simulink model "Model_1_PI_Gain_TestBench"  (R2021a)
settings: Solver=VariableStepAuto  StartTime=0.0  StopTime=5  MaxStep=1e-4  RelTol=1e-3  EnableMultiTasking=on
values from neighbouring files (symbols this model uses):
  Gain_I = 26    [Model_1_Initialization.m]
  Gain_P = 7    [Model_1_Initialization.m]
  Id_reference = 0    [Model_1_Initialization.m]
  Iq_reference = 100    [Model_1_Initialization.m]
  Lambda_m = 0.2205    [Model_1_Initialization.m]
  Ld = 1.7e-3    (= 0.0017)    [Model_1_Initialization.m]
  Lq = 3.2e-3    (= 0.0032)    [Model_1_Initialization.m]
  Polepairs = 4    [Model_1_Initialization.m]
  Rs = 0.02    [Model_1_Initialization.m]
libraries: spsSVPWMGenerator2LevelLib x6, spsControlledVoltageSourceLib x3, spsVoltageMeasurementLib x3, pid_lib x2, spsPermanentMagnetSynchronousMachineLib x1, spsGroundLib x1, spspowerguiLib x1
settings Model: Creator=dakaihu  LastModifiedBy=Hidayet
settings SolverCC: AlgebraicLoopSolver=TrustRegion
settings DataIOCC: LimitDataPoints=on  ReturnWorkspaceOutputs=off
settings OptimizationCC: LifeSpan=inf
settings DebuggingCC: AllowSymbolicDim=off  SFUnexpectedBacktrackingDiag=warning  SFNoUnconditionalDefaultTransitionDiag=warning  SFExecutionAtInitializationDiag=none  SFMachineParentedDataDiag=warning  ArithmeticOperatorsInVariantConditions=warning
settings ModelReferenceCC: PropagateSignalLabelsOutOfModel=off
settings SFSimCC: SimUseLocalCustomCode=off  CustomCodeUndefinedFunction=UseInterfaceOnly
settings RTWCC: RTWUseLocalCustomCode=off
settings CodeAppCC: StateflowObjectComments=on
settings GRTTargetCC: TargetLangStandard=C89/C90 (ANSI)
settings ConfigComp: CovMetricSettings=dw  CovSaveCumulativeToWorkspaceVar=on  CovSaveSingleToWorkspaceVar=on  CovExternalEMLEnable=off
settings SimscapeCC: SimscapeNormalizeSystem=off

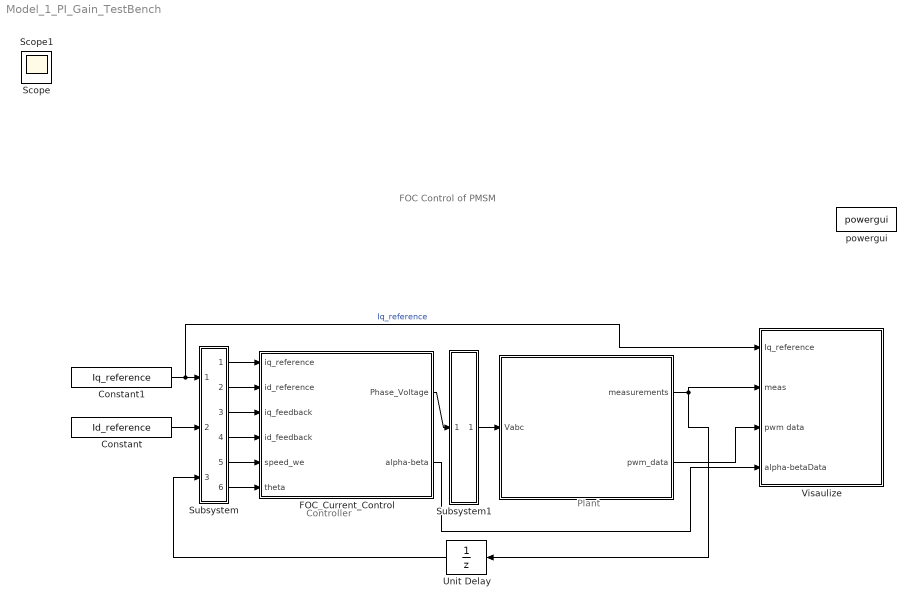
== system Model_1_PI_Gain_TestBench ==
  note: Controller
  note: Plant
  note: FOC Control of PMSM
  " " : Subsystem
  Constant : Constant  Value=Id_reference
  Constant1 : Constant  Value=Iq_reference  VectorParams1D=off
  FOC_Current_Control : Subsystem
  Subsystem : Subsystem
      mask Display: fprintf('C/D')
  Subsystem1 : Subsystem
      mask Display: fprintf('D/C')
  Unit Delay : UnitDelay  SampleTime=1e-4  HasFrameUpgradeWarning=on
  Visaulize : Subsystem
  powergui : spspowerguiLib/powergui  SimulationMode=Continuous  SampleTime=1e-5  frequency=60  Iterations=50  frequencyindice=0  Pbase=100e6  ErrMax=1e-4  UnitsV=kV  UnitsW=MW  buscounter=0  FunctionMessages=off  echomessages=off  EnableUseOfTLC=off  CurrentSourceSwitches=off  DisableSnubberDevices=off  DisableRonSwitches=off  DisableVfSwitches=off  DisplayEquations=off  AutomaticDiscreteSolvers=off  SolverType=Tustin/Backward Euler (TBE)  Interpol=off  ExternalGateDelay=off  methode=off  Ts=100  x0status=blocks  SPID=on  SwTol=0  HookPort=off  NonlinearTolerance=1e-4  nMaxIteration=100  ContinueOnMaxIteration=off  RestoreLinks=warning  ResistiveCurrentMeasurement=off  Frange=[0:2:500]  Ylog=off  Xlog=on  ShowGrid=off  save=off  variable=ZData  structure=0  ZoomFFT=on  StartTime=0.0  cycles=1  DisplayStyle=1  fundamental=60  FreqAxis=off  MaxFrequency=1000  frequencyindicesteady=1  RmsSteady=1  display=off
  Scope : Scope
  Scope1 : Scope
  wires:
  FOC_Current_Control/1(Phase_Voltage) -> Subsystem1/1(In1)
  " "/1(measurements) -> Unit Delay/1, Visaulize/2(meas)
  Subsystem/3(Out2) -> FOC_Current_Control/3(iq_feedback)
  Subsystem/4(Out3) -> FOC_Current_Control/4(id_feedback)
  Subsystem1/1(Out1) -> " "/1(Vabc)
  Unit Delay/1 -> Subsystem/3(PMSM_Measurements)
  Subsystem/5(Out1) -> FOC_Current_Control/5(speed_we)
  Subsystem/6(Out4) -> FOC_Current_Control/6(theta)
  Constant/1 -> Subsystem/2(id_ref)
  Constant1/1 -> Visaulize/1(Iq_reference), Subsystem/1(iq_ref)  "Iq_reference"
  Subsystem/1(Out6) -> FOC_Current_Control/1(iq_reference)
  Subsystem/2(Out5) -> FOC_Current_Control/2(id_reference)
  FOC_Current_Control/2(alpha-beta) -> Visaulize/4(alpha-betaData)
  " "/2(pwm_data) -> Visaulize/3(pwm data)

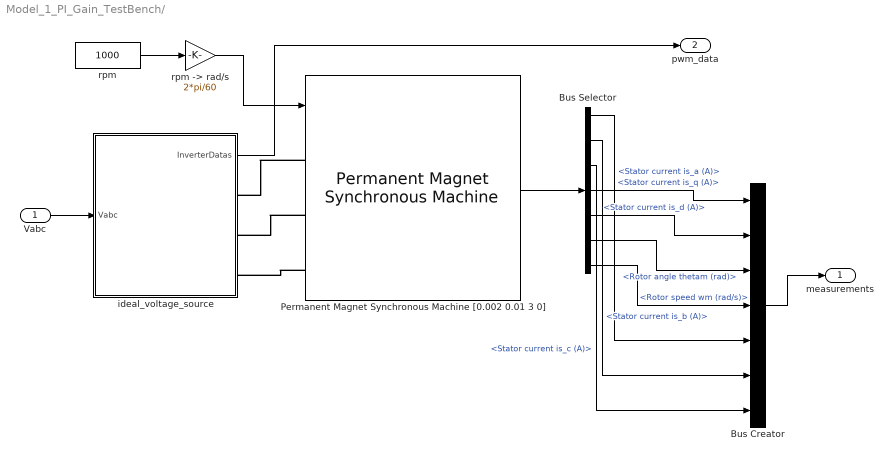
== system Model_1_PI_Gain_TestBench/  ==
  Vabc : Inport
  Bus Creator : BusCreator  Inputs=7
  Bus Selector : BusSelector  OutputSignals=Stator current is_a (A),Stator current is_b (A),Stator current is_c (A),Stator current is_q (A),Stator current is_d (A),Rotor angle thetam (rad),Rotor speed wm (rad/s)
  Permanent Magnet Synchronous Machine [0.002 0.01 3 0] : spsPermanentMagnetSynchronousMachineLib/Permanent Magnet Synchronous Machine  NbPhases=3  FluxDistribution=Sinusoidal  RotorType=Salient-pole  MechanicalLoad=Speed w  PresetModel=No  ShowDetailedParameters=on  MeasurementBus=off  Resistance=Rs  Inductance=8.5e-3  dqInductances=[Ld,Lq]  La=0.000395  MachineConstant=Flux linkage established by magnets (V.s)  Flux=Lambda_m  VoltageCst=159.9771  TorqueCst=1.323  Flat=120  Mechanical=[0.0027 0.001 4 0]  PolePairs=Polepairs  InitialConditions=[0,0, 0,0]  InitialConditions5ph=[0 0 0 0 0 0]  RefAngle=Aligned with phase A axis (original Park)  IterativeDiscreteModel=Trapezoidal non iterative  TsBlock=-1  TsPowergui=0
  ideal_voltage_source : Subsystem  VariantControl=variantPwm == enumPwm.behavior
  rpm : Constant  Value=1000
  "rpm -> rad/s" : Gain  Gain=2*pi/60
  measurements : Outport  VectorParamsAs1DForOutWhenUnconnected=off
  pwm_data : Outport  Port=2
  wires:
  Vabc/1 -> ideal_voltage_source/1(Vabc)
  rpm/1 -> "rpm -> rad/s"/1
  Bus Selector/4 -> Bus Creator/1  "<Stator current is_q (A)>"
  Bus Selector/5 -> Bus Creator/2  "<Stator current is_d (A)>"
  Bus Selector/6 -> Bus Creator/3  "<Rotor angle thetam (rad)>"
  Bus Creator/1 -> measurements/1
  Bus Selector/1 -> Bus Creator/5  "<Stator current is_a (A)>"
  Bus Selector/2 -> Bus Creator/6  "<Stator current is_b (A)>"
  Bus Selector/3 -> Bus Creator/7  "<Stator current is_c (A)>"
  Permanent Magnet Synchronous Machine [0.002 0.01 3 0]/1 -> Bus Selector/1
  Bus Selector/7 -> Bus Creator/4  "<Rotor speed wm (rad/s)>"
  "rpm -> rad/s"/1 -> Permanent Magnet Synchronous Machine [0.002 0.01 3 0]/1
  ideal_voltage_source/1(InverterDatas) -> pwm_data/1
  connections:
  Permanent Magnet Synchronous Machine [0.002 0.01 3 0]/LConn1 -- ideal_voltage_source/RConn1
  Permanent Magnet Synchronous Machine [0.002 0.01 3 0]/LConn2 -- ideal_voltage_source/RConn2
  Permanent Magnet Synchronous Machine [0.002 0.01 3 0]/LConn3 -- ideal_voltage_source/RConn3

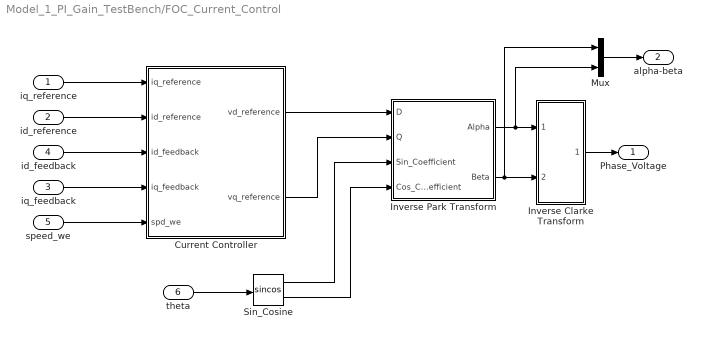
== system Model_1_PI_Gain_TestBench/FOC_Current_Control ==
  iq_reference : Inport  SampleTime=1e-4
  id_reference : Inport  Port=2  SampleTime=1e-4
  iq_feedback : Inport  Port=3  SampleTime=1e-4
  id_feedback : Inport  Port=4  SampleTime=1e-4
  speed_we : Inport  Port=5  SampleTime=1e-4
  theta : Inport  Port=6  SampleTime=1e-4
  Current Controller : Subsystem
  Inverse Clarke Transform : Subsystem
  Inverse Park Transform : Subsystem
  Mux : Mux  Inputs=2
  Sin_Cosine : Trigonometry  Operator=sincos
  Phase_Voltage : Outport  SampleTime=1e-4  VectorParamsAs1DForOutWhenUnconnected=off
  alpha-beta : Outport  Port=2
  wires:
  Inverse Clarke Transform/1(ABC) -> Phase_Voltage/1
  Sin_Cosine/2 -> Inverse Park Transform/4(Cos_Coefficient)
  Sin_Cosine/1 -> Inverse Park Transform/3(Sin_Coefficient)
  theta/1 -> Sin_Cosine/1
  Current Controller/2(vq_reference) -> Inverse Park Transform/2(Q)
  Current Controller/1(vd_reference) -> Inverse Park Transform/1(D)
  id_feedback/1 -> Current Controller/3(id_feedback)
  iq_feedback/1 -> Current Controller/4(iq_feedback)
  speed_we/1 -> Current Controller/5(spd_we)
  iq_reference/1 -> Current Controller/1(iq_reference)
  id_reference/1 -> Current Controller/2(id_reference)
  Mux/1 -> alpha-beta/1
  Inverse Park Transform/1(Alpha) -> Mux/2, Inverse Clarke Transform/1(Alpha)
  Inverse Park Transform/2(Beta) -> Mux/1, Inverse Clarke Transform/2(Beta)

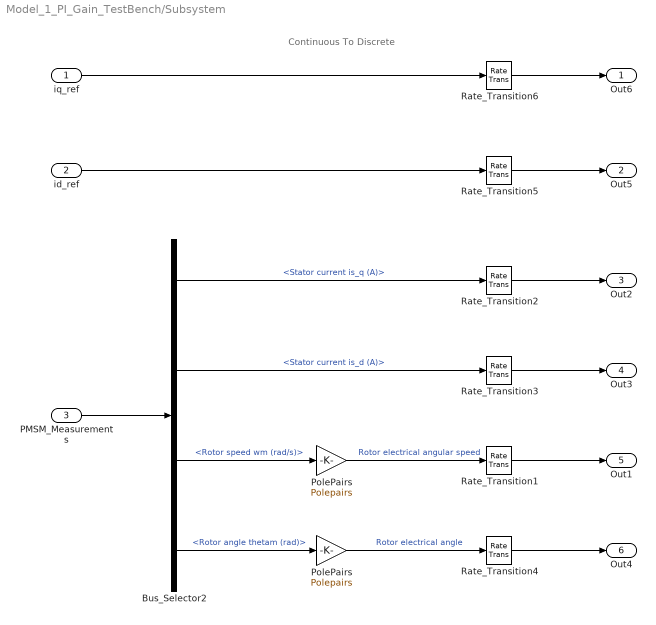
== system Model_1_PI_Gain_TestBench/Subsystem ==
  note: Continuous To Discrete
  iq_ref : Inport
  id_ref : Inport  Port=2
  PMSM_Measurements : Inport  Port=3
  Bus_Selector2 : BusSelector  OutputSignals=Stator current is_q (A),Stator current is_d (A),Rotor speed wm (rad/s),Rotor angle thetam (rad)
  PolePairs : Gain  Gain=Polepairs
  "PolePairs " : Gain  Gain=Polepairs
  Rate_Transition{1..6} (6 alike) : RateTransition  Integrity=off  Deterministic=off
  Out6 : Outport  VectorParamsAs1DForOutWhenUnconnected=off
  Out5 : Outport  Port=2  VectorParamsAs1DForOutWhenUnconnected=off
  Out2 : Outport  Port=3  VectorParamsAs1DForOutWhenUnconnected=off
  Out3 : Outport  Port=4  VectorParamsAs1DForOutWhenUnconnected=off
  Out1 : Outport  Port=5  VectorParamsAs1DForOutWhenUnconnected=off
  Out4 : Outport  Port=6  VectorParamsAs1DForOutWhenUnconnected=off
  wires:
  Rate_Transition4/1 -> Out4/1
  Bus_Selector2/2 -> Rate_Transition3/1  "<Stator current is_d (A)>"
  id_ref/1 -> Rate_Transition5/1
  iq_ref/1 -> Rate_Transition6/1
  Bus_Selector2/1 -> Rate_Transition2/1  "<Stator current is_q (A)>"
  Bus_Selector2/4 -> PolePairs/1  "<Rotor angle thetam (rad)>"
  PMSM_Measurements/1 -> Bus_Selector2/1
  PolePairs/1 -> Rate_Transition4/1  "Rotor electrical angle"
  Rate_Transition5/1 -> Out5/1
  Rate_Transition6/1 -> Out6/1
  Rate_Transition2/1 -> Out2/1
  Rate_Transition3/1 -> Out3/1
  Rate_Transition1/1 -> Out1/1
  Bus_Selector2/3 -> "PolePairs "/1  "<Rotor speed wm (rad/s)>"
  "PolePairs "/1 -> Rate_Transition1/1  "Rotor electrical angular speed"

== system Model_1_PI_Gain_TestBench/Subsystem1 ==
  In1 : Inport
  Rate_Transition1 : RateTransition  Integrity=off
  Out1 : Outport  VectorParamsAs1DForOutWhenUnconnected=off
  wires:
  In1/1 -> Rate_Transition1/1
  Rate_Transition1/1 -> Out1/1

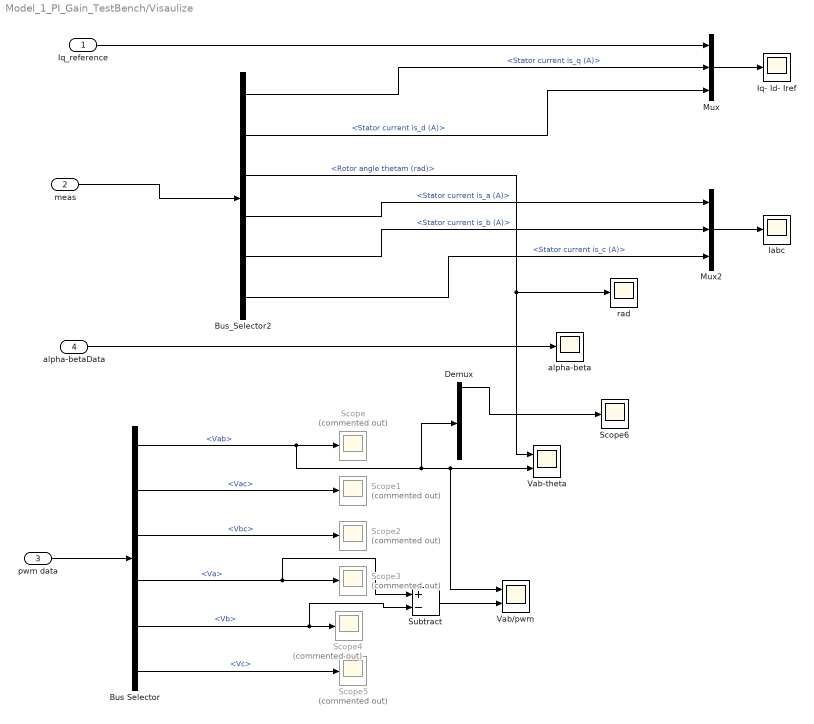
== system Model_1_PI_Gain_TestBench/Visaulize ==
  Iq_reference : Inport
  meas : Inport  Port=2
  pwm data : Inport  Port=3
  alpha-betaData : Inport  Port=4
  Bus Selector : BusSelector  OutputSignals=Vab,Vac,Vbc,Va,Vb,Vc
  Bus_Selector2 : BusSelector  OutputSignals=Stator current is_q (A),Stator current is_d (A),Rotor angle thetam (rad),Stator current is_a (A),Stator current is_b (A),Stator current is_c (A)
  Demux : Demux  Outputs=6
  Iabc : Scope
  Iq- Id- Iref : Scope
  Mux : Mux  Inputs=3
  Mux2 : Mux  Inputs=3
  Scope{,1..5} (6 alike) : Scope  Commented=on
  Scope6 : Scope
  Subtract : Sum  Inputs=+-
  Vab-theta : Scope  NumInputPorts=2
  Vab/pwm : Scope  NumInputPorts=2
  alpha-beta : Scope
  rad : Scope
  wires:
  meas/1 -> Bus_Selector2/1
  Mux/1 -> Iq- Id- Iref/1
  Bus_Selector2/2 -> Mux/3  "<Stator current is_d (A)>"
  Iq_reference/1 -> Mux/1
  Bus_Selector2/1 -> Mux/2  "<Stator current is_q (A)>"
  Mux2/1 -> Iabc/1
  alpha-betaData/1 -> alpha-beta/1
  Bus_Selector2/3 -> Vab-theta/1, rad/1  "<Rotor angle thetam (rad)>"
  pwm data/1 -> Bus Selector/1
  Bus Selector/1 -> Demux/1, Vab/pwm/1, Vab-theta/2, Scope/1  "<Vab>"
  Bus Selector/2 -> Scope1/1  "<Vac>"
  Bus Selector/3 -> Scope2/1  "<Vbc>"
  Bus Selector/4 -> Subtract/1, Scope3/1  "<Va>"
  Bus Selector/5 -> Subtract/2, Scope4/1  "<Vb>"
  Subtract/1 -> Vab/pwm/2
  Bus Selector/6 -> Scope5/1  "<Vc>"
  Bus_Selector2/4 -> Mux2/1  "<Stator current is_a (A)>"
  Bus_Selector2/5 -> Mux2/2  "<Stator current is_b (A)>"
  Bus_Selector2/6 -> Mux2/3  "<Stator current is_c (A)>"
  Demux/1 -> Scope6/1

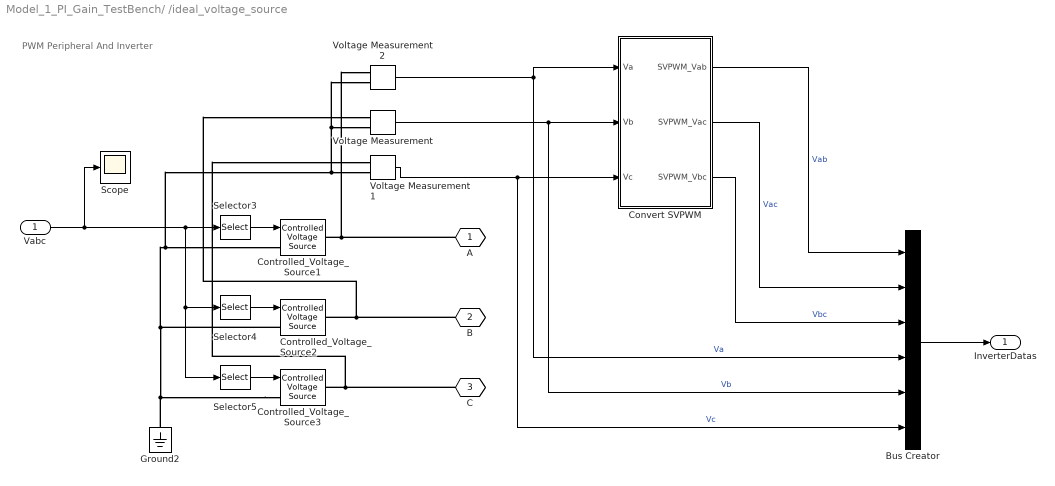
== system Model_1_PI_Gain_TestBench/ /ideal_voltage_source ==
  note: PWM Peripheral And Inverter
  Vabc : Inport
  Bus Creator : BusCreator  Inputs=6
  Controlled_Voltage_Source1 : spsControlledVoltageSourceLib/Controlled Voltage Source  Initialize=off  Source_Type=DC  Amplitude=12  Phase=0  Frequency=0  Measurements=None
  Controlled_Voltage_Source2 : spsControlledVoltageSourceLib/Controlled Voltage Source  Initialize=off  Source_Type=DC  Amplitude=12  Phase=0  Frequency=0  Measurements=None
  Controlled_Voltage_Source3 : spsControlledVoltageSourceLib/Controlled Voltage Source  Initialize=off  Source_Type=DC  Amplitude=12  Phase=0  Frequency=0  Measurements=None
  Convert SVPWM : Subsystem
  Ground2 : spsGroundLib/Ground  LConnTagsString=a
  Scope : Scope
  Selector3 : Selector  InputPortWidth=3  IndexOptions=Index vector (dialog)  Indices=[1]  OutputSizes=1
  Selector4 : Selector  InputPortWidth=3  IndexOptions=Index vector (dialog)  Indices=2  OutputSizes=1
  Selector5 : Selector  InputPortWidth=3  IndexOptions=Index vector (dialog)  Indices=3  OutputSizes=1
  Voltage Measurement : spsVoltageMeasurementLib/Voltage Measurement  PhasorSimulation=off  OutputType=Complex  PSBequivalent=0
  Voltage Measurement1 : spsVoltageMeasurementLib/Voltage Measurement  PhasorSimulation=off  OutputType=Complex  PSBequivalent=0
  Voltage Measurement2 : spsVoltageMeasurementLib/Voltage Measurement  PhasorSimulation=off  OutputType=Complex  PSBequivalent=0
  A : PMIOPort  Tag=PMCPort  Side=Right
  B : PMIOPort  Tag=PMCPort  Port=2  Side=Right
  C : PMIOPort  Tag=PMCPort  Port=3  Side=Right
  InverterDatas : Outport
  wires:
  Vabc/1 -> Scope/1, Selector4/1, Selector5/1, Selector3/1
  Selector5/1 -> Controlled_Voltage_Source3/1
  Selector4/1 -> Controlled_Voltage_Source2/1
  Selector3/1 -> Controlled_Voltage_Source1/1
  Voltage Measurement2/1 -> Bus Creator/4, Convert SVPWM/1(Va)  "Va"
  Voltage Measurement/1 -> Bus Creator/5, Convert SVPWM/2(Vb)  "Vb"
  Voltage Measurement1/1 -> Bus Creator/6, Convert SVPWM/3(Vc)  "Vc"
  Convert SVPWM/1(SVPWM_Vab) -> Bus Creator/1  "Vab"
  Convert SVPWM/2(SVPWM_Vac) -> Bus Creator/2  "Vac"
  Convert SVPWM/3(SVPWM_Vbc) -> Bus Creator/3  "Vbc"
  Bus Creator/1 -> InverterDatas/1
  connections:
  C/RConn1 -- Voltage Measurement1/LConn1 -- Controlled_Voltage_Source3/RConn1
  B/RConn1 -- Voltage Measurement/LConn1 -- Controlled_Voltage_Source2/RConn1
  A/RConn1 -- Voltage Measurement2/LConn1 -- Controlled_Voltage_Source1/RConn1
  Controlled_Voltage_Source3/LConn1 -- Voltage Measurement2/LConn2 -- Voltage Measurement/LConn2 -- Voltage Measurement1/LConn2 -- Controlled_Voltage_Source1/LConn1 -- Controlled_Voltage_Source2/LConn1 -- Ground2/LConn1

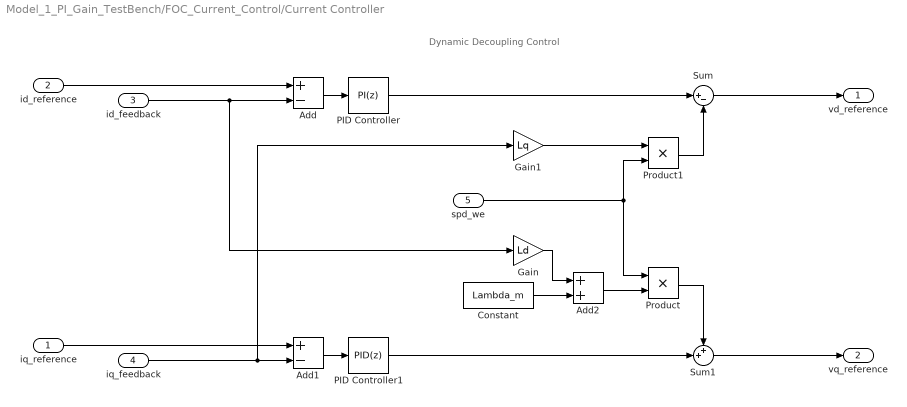
== system Model_1_PI_Gain_TestBench/FOC_Current_Control/Current Controller ==
  note: Dynamic Decoupling Control
  iq_reference : Inport  SampleTime=1e-4
  id_reference : Inport  Port=2  SampleTime=1e-4
  id_feedback : Inport  Port=3  SampleTime=1e-4
  iq_feedback : Inport  Port=4  SampleTime=1e-4
  spd_we : Inport  Port=5  SampleTime=1e-4
  Add : Sum  Inputs=+-
  Add1 : Sum  Inputs=+-
  Add2 : Sum
  Constant : Constant  Value=Lambda_m  SampleTime=1e-4
  Gain : Gain  Gain=Ld
  Gain1 : Gain  Gain=Lq
  PID Controller : pid_lib/PID Controller  Controller=PI  Form=Parallel  TimeDomain=Discrete-time  UseExternalTs=off  SampleTime=-1  IntegratorMethod=Forward Euler  FilterMethod=Forward Euler  ControllerParametersSource=internal  P=Gain_P  I=Gain_I  D=0  UseFilter=on  N=100  TunerSelectOption=Transfer Function Based (PID Tuner App)  InitialConditionSource=internal  InitialConditionForIntegrator=0  InitialConditionForFilter=0  DifferentiatorICPrevScaledInput=0  ExternalReset=none  TrackingMode=off  Kt=1  LimitOutput=off  SatLimitsSource=internal  UpperSaturationLimit=inf  LowerSaturationLimit=-inf  LinearizeAsGain=on  AntiWindupMode=none  Kb=1  POutMin=[]  POutMax=[]  IOutMin=[]  IOutMax=[]  DOutMin=[]  DOutMax=[]  NOutMin=[]  NOutMax=[]  SumOutMin=[]  SumOutMax=[]  SaturationOutMin=[]  SaturationOutMax=[]  PParamMin=[]  PParamMax=[]  IParamMin=[]  IParamMax=[]  DParamMin=[]  DParamMax=[]  NParamMin=[]  NParamMax=[]  KbParamMin=[]  KbParamMax=[]  KtParamMin=[]  KtParamMax=[]  KbOutMin=[]  KbOutMax=[]  KtOutMin=[]  KtOutMax=[]  IntegratorOutMin=[]  IntegratorOutMax=[]  FilterOutMin=[]  FilterOutMax=[]  SumI1OutMin=[]  SumI1OutMax=[]  SumI2OutMin=[]  SumI2OutMax=[]  SumI3OutMin=[]  SumI3OutMax=[]  SumI4OutMin=[]  SumI4OutMax=[]  SumDOutMin=[]  SumDOutMax=[]  DifferentiatorOutMin=[]  DifferentiatorOutMax=[]  FilterDiffOutCoefMin=[]  FilterDiffOutCoefMax=[]  ReciprocalOutMin=[]  ReciprocalOutMax=[]  SumDenOutMin=[]  SumDenOutMax=[]  SumNumOutMin=[]  SumNumOutMax=[]  DivideOutMin=[]  DivideOutMax=[]  UdiffTsProdOutMin=[]  UdiffTsProdOutMax=[]  NTsProdOutMin=[]  NTsProdOutMax=[]  UintegralTsProdOutMin=[]  UintegralTsProdOutMax=[]  UngainTsProdOutMin=[]  UngainTsProdOutMax=[]  IntegratorContinuousStateAttributes=''  IntegratorStateMustResolveToSignalObject=off  IntegratorRTWStateStorageClass=Auto  FilterContinuousStateAttributes=''  FilterStateMustResolveToSignalObject=off  FilterRTWStateStorageClass=Auto  ParallelPVariant=InternalParameters  IdealPVariant=Disabled  IVariant=InternalParameters  DVariant=Disabled  IntegratorVariant=Discrete  SatVariant=Disabled  AWVariant=Passthrough  PCopyVariant=Disabled  TRVariant=Disabled  FdbkBlocksVariant=Forward  IdealPFdbkVariant=Disabled  SatFdbkVariant=Disabled  DerivativeFilterVariant=Disabled  NVariant=Disabled  NCopyVariant=Disabled_SignalSpec  FilterICVariant=Disabled  IntegratorICVariant=InternalICs  ExternalResetVariant=Disabled  TRSumVariant=Passthrough  SumFdbkVariant=Disabled  SumVariant=Sum_PI  TsampFilterVariant=InternalTs  TsampNgainVariant=Passthrough  TsampIntegralVariant=Passthrough  ExternalSaturationOutDataTypeStr=Inherit: Same as second input
  PID Controller1 : pid_lib/PID Controller  Controller=PID  Form=Parallel  TimeDomain=Discrete-time  UseExternalTs=off  SampleTime=-1  IntegratorMethod=Forward Euler  FilterMethod=Forward Euler  ControllerParametersSource=internal  P=Gain_P  I=Gain_I  D=0  UseFilter=on  N=100  TunerSelectOption=Transfer Function Based (PID Tuner App)  InitialConditionSource=internal  InitialConditionForIntegrator=0  InitialConditionForFilter=0  DifferentiatorICPrevScaledInput=0  ExternalReset=none  TrackingMode=off  Kt=1  LimitOutput=off  SatLimitsSource=internal  UpperSaturationLimit=inf  LowerSaturationLimit=-inf  LinearizeAsGain=on  AntiWindupMode=none  Kb=1  POutMin=[]  POutMax=[]  IOutMin=[]  IOutMax=[]  DOutMin=[]  DOutMax=[]  NOutMin=[]  NOutMax=[]  SumOutMin=[]  SumOutMax=[]  SaturationOutMin=[]  SaturationOutMax=[]  PParamMin=[]  PParamMax=[]  IParamMin=[]  IParamMax=[]  DParamMin=[]  DParamMax=[]  NParamMin=[]  NParamMax=[]  KbParamMin=[]  KbParamMax=[]  KtParamMin=[]  KtParamMax=[]  KbOutMin=[]  KbOutMax=[]  KtOutMin=[]  KtOutMax=[]  IntegratorOutMin=[]  IntegratorOutMax=[]  FilterOutMin=[]  FilterOutMax=[]  SumI1OutMin=[]  SumI1OutMax=[]  SumI2OutMin=[]  SumI2OutMax=[]  SumI3OutMin=[]  SumI3OutMax=[]  SumI4OutMin=[]  SumI4OutMax=[]  SumDOutMin=[]  SumDOutMax=[]  DifferentiatorOutMin=[]  DifferentiatorOutMax=[]  FilterDiffOutCoefMin=[]  FilterDiffOutCoefMax=[]  ReciprocalOutMin=[]  ReciprocalOutMax=[]  SumDenOutMin=[]  SumDenOutMax=[]  SumNumOutMin=[]  SumNumOutMax=[]  DivideOutMin=[]  DivideOutMax=[]  UdiffTsProdOutMin=[]  UdiffTsProdOutMax=[]  NTsProdOutMin=[]  NTsProdOutMax=[]  UintegralTsProdOutMin=[]  UintegralTsProdOutMax=[]  UngainTsProdOutMin=[]  UngainTsProdOutMax=[]  IntegratorContinuousStateAttributes=''  IntegratorStateMustResolveToSignalObject=off  IntegratorRTWStateStorageClass=Auto  FilterContinuousStateAttributes=''  FilterStateMustResolveToSignalObject=off  FilterRTWStateStorageClass=Auto  ParallelPVariant=InternalParameters  IdealPVariant=Disabled  IVariant=InternalParameters  DVariant=InternalParameters  IntegratorVariant=Discrete  SatVariant=Disabled  AWVariant=Passthrough  PCopyVariant=Disabled  TRVariant=Disabled  FdbkBlocksVariant=Forward  IdealPFdbkVariant=Disabled  SatFdbkVariant=Disabled  DerivativeFilterVariant=ForwardEulerFilter  NVariant=InternalParameters  NCopyVariant=Disabled  FilterICVariant=InternalICsFilter  IntegratorICVariant=InternalICs  ExternalResetVariant=Disabled  TRSumVariant=Passthrough  SumFdbkVariant=Disabled  SumVariant=Sum_PID  TsampFilterVariant=InternalTs  TsampNgainVariant=Passthrough  TsampIntegralVariant=Passthrough  ExternalSaturationOutDataTypeStr=Inherit: Same as second input
  Product : Product
  Product1 : Product
  Sum : Sum  Inputs=|+-
  Sum1 : Sum  Inputs=++|
  vd_reference : Outport  SampleTime=1e-4  VectorParamsAs1DForOutWhenUnconnected=off
  vq_reference : Outport  Port=2  SampleTime=1e-4  VectorParamsAs1DForOutWhenUnconnected=off
  wires:
  Sum/1 -> vd_reference/1
  PID Controller/1 -> Sum/1
  id_feedback/1 -> Gain/1, Add/2
  Add/1 -> PID Controller/1
  iq_feedback/1 -> Gain1/1, Add1/2
  id_reference/1 -> Add/1
  Add1/1 -> PID Controller1/1
  iq_reference/1 -> Add1/1
  Sum1/1 -> vq_reference/1
  PID Controller1/1 -> Sum1/2
  Gain/1 -> Add2/1
  Constant/1 -> Add2/2
  Add2/1 -> Product/2
  spd_we/1 -> Product1/2, Product/1
  Gain1/1 -> Product1/1
  Product1/1 -> Sum/2
  Product/1 -> Sum1/1

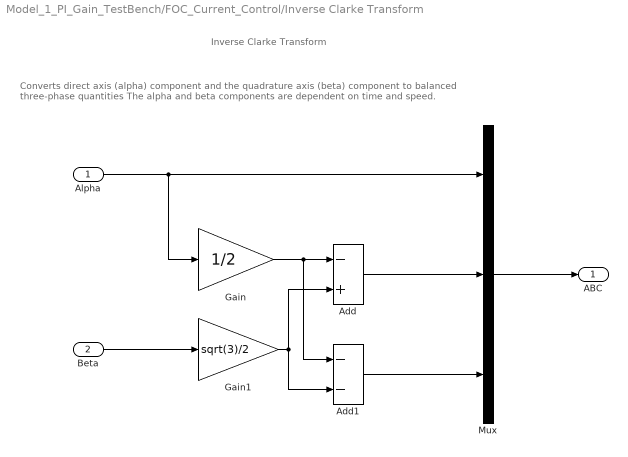
== system Model_1_PI_Gain_TestBench/FOC_Current_Control/Inverse Clarke Transform ==
  note: Inverse Clarke Transform
  note: Converts direct axis (alpha) component and the quadrature axis (beta) component to balanced three-phase quantities
      | The alpha and beta components are dependent on time and speed.
  Alpha : Inport
  Beta : Inport  Port=2
  Add : Sum  Inputs=-+  OutDataTypeStr=Inherit: Same as first input
  Add1 : Sum  Inputs=--  OutDataTypeStr=Inherit: Same as first input
  Gain : Gain  Gain=1/2
  Gain1 : Gain  Gain=sqrt(3)/2
  Mux : Mux  Inputs=3
  ABC : Outport  VectorParamsAs1DForOutWhenUnconnected=off
  wires:
  Beta/1 -> Gain1/1
  Mux/1 -> ABC/1
  Alpha/1 -> Mux/1, Gain/1
  Add1/1 -> Mux/3
  Gain1/1 -> Add1/2, Add/2
  Gain/1 -> Add1/1, Add/1
  Add/1 -> Mux/2

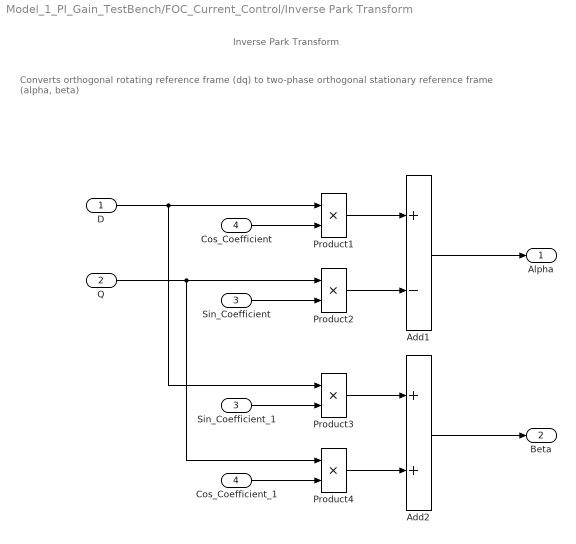
== system Model_1_PI_Gain_TestBench/FOC_Current_Control/Inverse Park Transform ==
  note: Converts orthogonal rotating reference frame (dq) to two-phase orthogonal stationary reference frame (alpha, beta)
  note: Inverse Park Transform
  D : Inport
  Q : Inport  Port=2
  Sin_Coefficient : Inport  Port=3
  Cos_Coefficient : Inport  Port=4
  Add1 : Sum  Inputs=+-  OutDataTypeStr=Inherit: Same as first input
  Add2 : Sum  OutDataTypeStr=Inherit: Same as first input
  Cos_Coefficient_1 : InportShadow  Port=4
  Product{1..4} (4 alike) : Product  RndMeth=Simplest
  Sin_Coefficient_1 : InportShadow  Port=3
  Alpha : Outport  VectorParamsAs1DForOutWhenUnconnected=off
  Beta : Outport  Port=2  VectorParamsAs1DForOutWhenUnconnected=off
  wires:
  Sin_Coefficient_1/1 -> Product3/2
  Product2/1 -> Add1/2
  Cos_Coefficient_1/1 -> Product4/2
  Add2/1 -> Beta/1
  Product3/1 -> Add2/1
  Add1/1 -> Alpha/1
  Product1/1 -> Add1/1
  Product4/1 -> Add2/2
  Sin_Coefficient/1 -> Product2/2
  D/1 -> Product3/1, Product1/1
  Q/1 -> Product2/1, Product4/1
  Cos_Coefficient/1 -> Product1/2

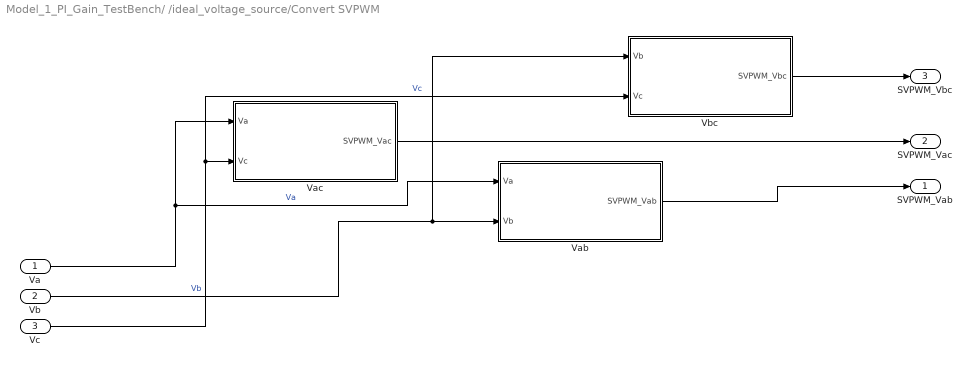
== system Model_1_PI_Gain_TestBench/ /ideal_voltage_source/Convert SVPWM ==
  Va : Inport
  Vb : Inport  Port=2
  Vc : Inport  Port=3
  Vab : Subsystem
  Vac : Subsystem
  Vbc : Subsystem
  SVPWM_Vab : Outport
  SVPWM_Vac : Outport  Port=2
  SVPWM_Vbc : Outport  Port=3
  wires:
  Vab/1(SVPWM_Vab) -> SVPWM_Vab/1
  Vac/1(SVPWM_Vac) -> SVPWM_Vac/1
  Vbc/1(SVPWM_Vbc) -> SVPWM_Vbc/1
  Va/1 -> Vab/1(Va), Vac/1(Va)  "Va"
  Vb/1 -> Vbc/1(Vb), Vab/2(Vb)  "Vb"
  Vc/1 -> Vbc/2(Vc), Vac/2(Vc)  "Vc"

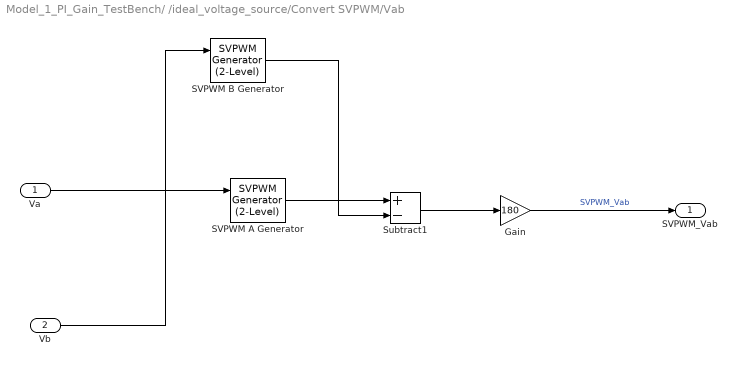
== system Model_1_PI_Gain_TestBench/ /ideal_voltage_source/Convert SVPWM/Vab ==
  Va : Inport
  Vb : Inport  Port=2
  Gain : Gain  Gain=180
  SVPWM A Generator : spsSVPWMGenerator2LevelLib/SVPWM Generator (2-Level)  InputType=Magnitude-Angle (rad)  SwitchingPattern=Pattern #1  Fc=2000  ParUref=[0.8 -30 50]  Ts=0
      settings: SourceProductBaseCode=PS
  SVPWM B Generator : spsSVPWMGenerator2LevelLib/SVPWM Generator (2-Level)  InputType=Magnitude-Angle (rad)  SwitchingPattern=Pattern #1  Fc=2000  ParUref=[0.8 120 50]  Ts=0
      settings: SourceProductBaseCode=PS
  Subtract1 : Sum  Inputs=+-
  SVPWM_Vab : Outport
  wires:
  SVPWM B Generator/1 -> Subtract1/2
  Gain/1 -> SVPWM_Vab/1  "SVPWM_Vab"
  Va/1 -> SVPWM A Generator/1
  Subtract1/1 -> Gain/1
  SVPWM A Generator/1 -> Subtract1/1
  Vb/1 -> SVPWM B Generator/1

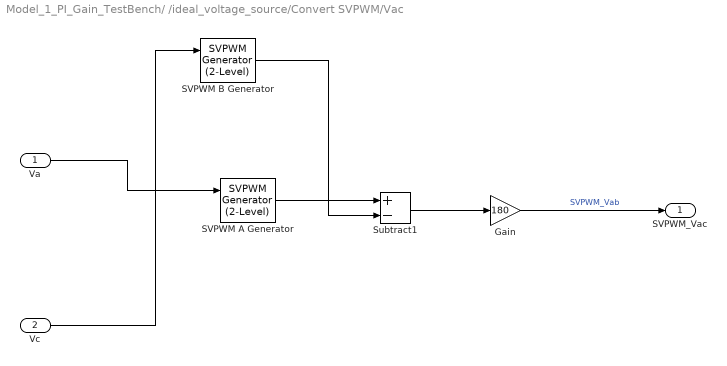
== system Model_1_PI_Gain_TestBench/ /ideal_voltage_source/Convert SVPWM/Vac ==
  Va : Inport
  Vc : Inport  Port=2
  Gain : Gain  Gain=180
  SVPWM A Generator : spsSVPWMGenerator2LevelLib/SVPWM Generator (2-Level)  InputType=Magnitude-Angle (rad)  SwitchingPattern=Pattern #1  Fc=2000  ParUref=[0.8 -30 50]  Ts=0
      settings: SourceProductBaseCode=PS
  SVPWM B Generator : spsSVPWMGenerator2LevelLib/SVPWM Generator (2-Level)  InputType=Magnitude-Angle (rad)  SwitchingPattern=Pattern #1  Fc=2000  ParUref=[0.8 120 50]  Ts=0
      settings: SourceProductBaseCode=PS
  Subtract1 : Sum  Inputs=+-
  SVPWM_Vac : Outport
  wires:
  SVPWM B Generator/1 -> Subtract1/2
  Gain/1 -> SVPWM_Vac/1  "SVPWM_Vab"
  Va/1 -> SVPWM A Generator/1
  Subtract1/1 -> Gain/1
  SVPWM A Generator/1 -> Subtract1/1
  Vc/1 -> SVPWM B Generator/1

== system Model_1_PI_Gain_TestBench/ /ideal_voltage_source/Convert SVPWM/Vbc ==
  Vb : Inport
  Vc : Inport  Port=2
  Gain : Gain  Gain=180
  SVPWM A Generator : spsSVPWMGenerator2LevelLib/SVPWM Generator (2-Level)  InputType=Magnitude-Angle (rad)  SwitchingPattern=Pattern #1  Fc=2000  ParUref=[0.8 -30 50]  Ts=0
      settings: SourceProductBaseCode=PS
  SVPWM B Generator : spsSVPWMGenerator2LevelLib/SVPWM Generator (2-Level)  InputType=Magnitude-Angle (rad)  SwitchingPattern=Pattern #1  Fc=2000  ParUref=[0.8 120 50]  Ts=0
      settings: SourceProductBaseCode=PS
  Subtract1 : Sum  Inputs=+-
  SVPWM_Vbc : Outport
  wires:
  Vc/1 -> SVPWM B Generator/1
  SVPWM A Generator/1 -> Subtract1/1
  Subtract1/1 -> Gain/1
  Vb/1 -> SVPWM A Generator/1
  Gain/1 -> SVPWM_Vbc/1  "SVPWM_Vab"
  SVPWM B Generator/1 -> Subtract1/2
